simulink model "Cessna_Model"  (R2023a)
settings: Solver=ode45  StartTime=0.0  StopTime=200  RelTol=1e-3
libraries: airlib x1
settings Model: Creator=Luca  LastModifiedBy=fraco
settings OptimizationCC: ReuseModelBlockBuffer=off

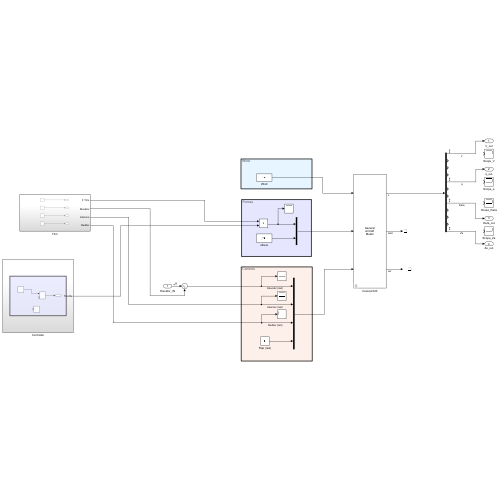
[thumbnail: Simulink's stored preview of the top-level diagram]
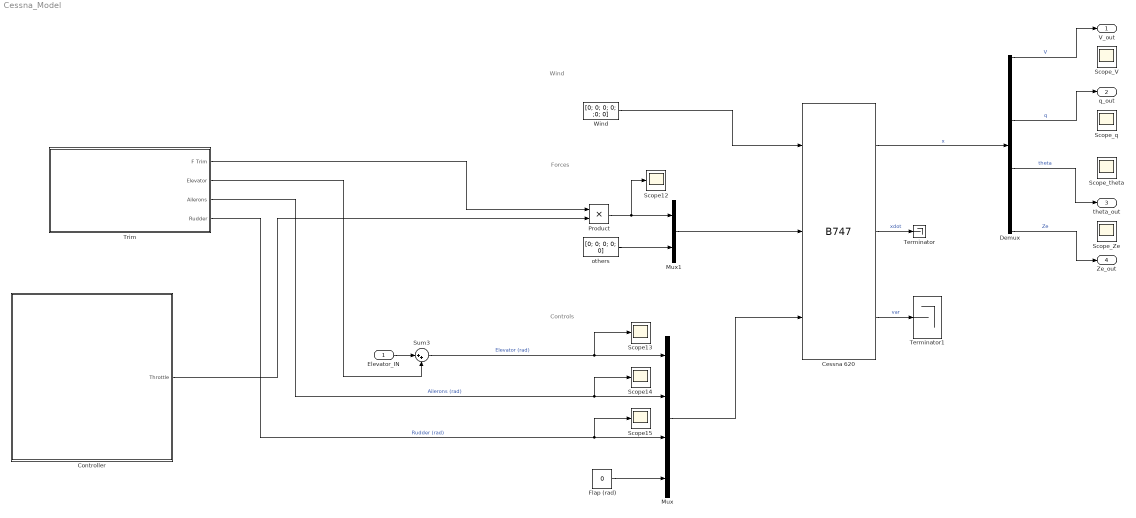
== system Cessna_Model ==
  note: Forces
  note: Controls
  note: Wind
  Elevator_IN : Inport
  " Cessna 620 " : airlib/B747  GM1="[2.006  16.7945  31.587  87872  23456  87509  0 0 0   6804]"  CD_wind="[0.0322   0.269  0  0  0]"  CL_wind="[0.48   5.55    7.5   0.58   0]"  Cm_body="[0.06  -1.18   -22.4   -1.73  0]"  CY_body="[0  -0.883  -0.227  0.448  0.0  0.2]"  Cl_body="[0   -0.1381  -0.566  0.1166  -0.1776  0.02]"  Cn_body="[0    0.1739   -0.0501   -0.2  0.0194  -0.1054]"  x0="[115  -0.0445 0   0 0 0   0 -0.0445 0   0 0 350]"
  Controller : Subsystem
  Demux : Demux  Outputs=12
  Flap (rad) : Constant  Value=0
  Mux : Mux
  Mux1 : Mux  Inputs=2
  Product : Product
  Scope{12..15} (4 alike) : Scope
  Scope_V : Scope
  Scope_Ze : Scope
  Scope_q : Scope
  Scope_theta : Scope
  Sum3 : Sum  Inputs=|++
  Terminator : Terminator
  Terminator1 : Terminator
  Trim : Subsystem
  Wind : Constant  Value=[0; 0; 0; 0; ;0; 0]
  others : Constant  Value=[0; 0; 0; 0; 0]
  V_out : Outport
  q_out : Outport  Port=2
  theta_out : Outport  Port=3
  Ze_out : Outport  Port=4
  wires:
  Demux/1 -> V_out/1  "V"
  Demux/5 -> q_out/1  "q"
  Demux/8 -> theta_out/1  "theta"
  Demux/12 -> Ze_out/1  "Ze"
  Flap (rad)/1 -> Mux/4
  others/1 -> Mux1/2
  " Cessna 620 "/1 -> Demux/1  "x"
  " Cessna 620 "/2 -> Terminator/1  "xdot"
  " Cessna 620 "/3 -> Terminator1/1  "var"
  Wind/1 -> " Cessna 620 "/1
  Mux1/1 -> " Cessna 620 "/2
  Mux/1 -> " Cessna 620 "/3
  Trim/4(Rudder) -> Scope15/1, Mux/3  "Rudder (rad)"
  Trim/3(Ailerons) -> Scope14/1, Mux/2  "Ailerons (rad)"
  Sum3/1 -> Mux/1, Scope13/1  "Elevator (rad)"
  Product/1 -> Scope12/1, Mux1/1
  Controller/1(Throttle) -> Product/2
  Trim/1(F Trim) -> Product/1
  Elevator_IN/1 -> Sum3/1
  Trim/2(Elevator) -> Sum3/2

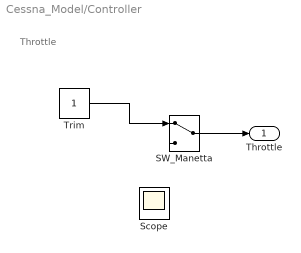
== system Cessna_Model/Controller ==
  note: Throttle
  SW_Manetta : ManualSwitch
  Scope : Scope
  Trim : Constant
  Throttle : Outport
  wires:
  Trim/1 -> SW_Manetta/1
  SW_Manetta/1 -> Throttle/1

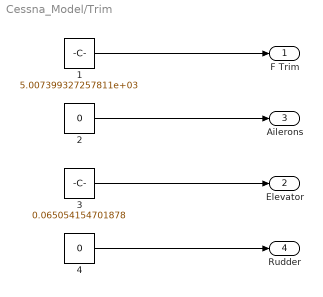
== system Cessna_Model/Trim ==
  1 : Constant  Value=5.007399327257811e+03
  2 : Constant  Value=0
  3 : Constant  Value=0.065054154701878
  4 : Constant  Value=0
  F Trim : Outport
  Elevator : Outport  Port=2
  Ailerons : Outport  Port=3
  Rudder : Outport  Port=4
  wires:
  1/1 -> F Trim/1
  2/1 -> Ailerons/1
  3/1 -> Elevator/1
  4/1 -> Rudder/1
